simulink model "arduino_encoder_2018a"  (R2018a)
settings: Solver=FixedStepDiscrete  StartTime=0.0  StopTime=inf  FixedStep=0.001  RelTol=1e-3  EnableMultiTasking=on
libraries: arduinolib x2
settings Model: SimulationMode=external  ExtModeTrigDuration=2  Creator=jedsada-emertxe  LastModifiedBy=jedsada-emertxe
settings SolverCC: AutoInsertRateTranBlk=on
settings OptimizationCC: EnhancedBackFolding=on  PassReuseOutputArgsAs=Individual arguments  MaxStackSize=64  OptimizeBlockOrder=speed  DifferentSizesBufferReuse=on  OptimizationCustomize=off
settings DebuggingCC: ParameterTunabilityLossMsg=error
settings HardwareCC: ProdBitPerInt=16  ProdBitPerPointer=16  ProdBitPerSizeT=16  ProdBitPerPtrDiffT=16  ProdLargestAtomicFloat=None  ProdWordSize=8  ProdHWDeviceType=Atmel->AVR
settings SFSimCC: MATLABDynamicMemAlloc=off
settings RTWCC: SystemTargetFile=ert.tlc  HardwareBoard=Arduino Uno  TLCOptions=-aInlineSetEventsForThisBaseRateFcn=TLC_FALSE -aSuppressMultiTaskScheduler=TLC_FALSE -aRateBasedStepFcn=1  TemplateMakefile=ert_default_tmf  GenerateReport=on  Toolchain=Arduino AVR  BuildConfiguration=Faster Runs  IncludeHyperlinkInReport=on  LaunchReport=on  GenerateTraceInfo=on  GenerateTraceReport=on  GenerateTraceReportSl=on  GenerateTraceReportSf=on  GenerateTraceReportEml=on
settings CodeAppCC: ForceParamTrailComments=on  IgnoreCustomStorageClasses=off  OperatorAnnotations=on  SimulinkDataObjDesc=on  SFDataObjDesc=on  InsertBlockDesc=on
settings ERTTargetCC: SupportContinuousTime=on  SupportVariableSizeSignals=on

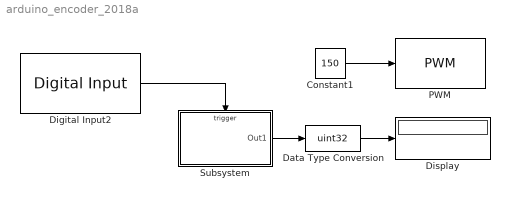
== system arduino_encoder_2018a ==
  Constant1 : Constant  Value=150
  Data Type Conversion : DataTypeConversion  OutDataTypeStr=uint32  ConvertRealWorld=Stored Integer (SI)  RndMeth=Round  SaturateOnIntegerOverflow=on
  Digital Input2 : arduinolib/Digital Input  pinNumber=2  sampleTime=0.001  blockPlatform=arduino
      settings: SourceProductName=Simulink Support Package for Arduino Hardware
  Display : Display
  PWM : arduinolib/PWM  pinNumber=6  EnableInputFrequency=off  InitialFrequency=2000  InitialDutyCycle=0  NotificationType=None  blockPlatform=arduino
  Subsystem : Subsystem
  wires:
  Constant1/1 -> PWM/1
  Digital Input2/1 -> Subsystem/Trigger
  Subsystem/1(Out1) -> Data Type Conversion/1
  Data Type Conversion/1 -> Display/1

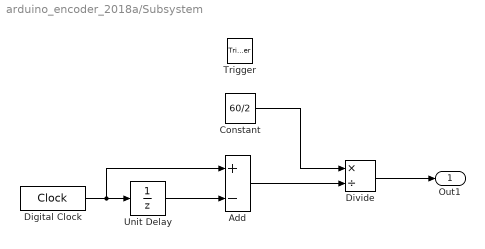
== system arduino_encoder_2018a/Subsystem ==
  Trigger : TriggerPort  VariantControl=Variant  InitialTriggerSignalState=positive  PortDimensions=1
  Add : Sum  Inputs=+-  RndMeth=Zero  SaturateOnIntegerOverflow=on
  Constant : Constant  Value=60/2  SampleTime=-1
  Digital Clock : DigitalClock  SampleTime=-1
  Divide : Product  Inputs=*/
  Unit Delay : UnitDelay  SampleTime=-1
  Out1 : Outport
  wires:
  Divide/1 -> Out1/1
  Add/1 -> Divide/2
  Constant/1 -> Divide/1
  Digital Clock/1 -> Add/1, Unit Delay/1
  Unit Delay/1 -> Add/2
